simulink model "lcl_filter"  (R2022b)
settings: Solver=VariableStepAuto  StartTime=0.0  StopTime=10.0  RelTol=1e-3
libraries: spsSeriesRLCBranchLib x3, spsCurrentMeasurementLib x1, spsVoltageMeasurementLib x1
settings Model: Creator=nisha  LastModifiedBy=nisha

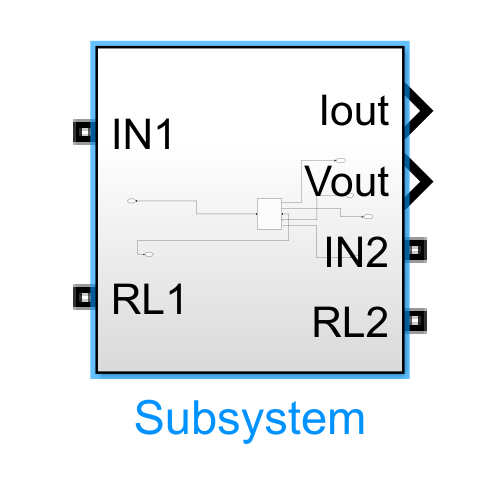
[thumbnail: Simulink's stored preview of the top-level diagram]
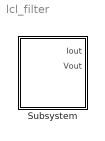
== system lcl_filter ==
  Subsystem : Subsystem

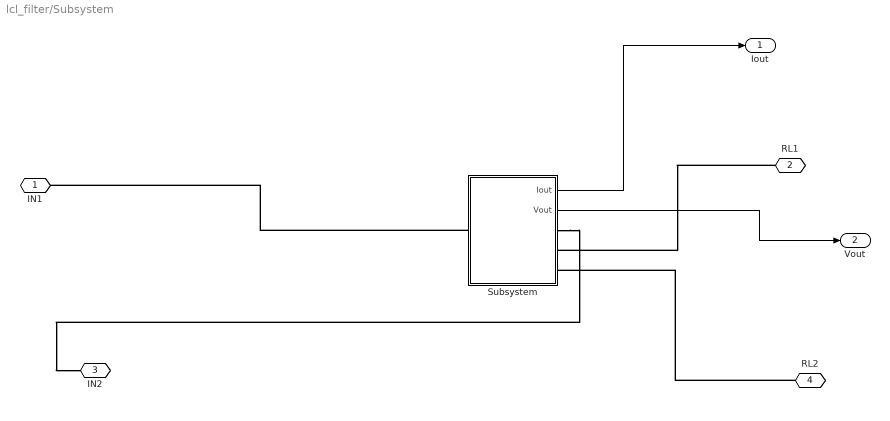
== system lcl_filter/Subsystem ==
  Subsystem : Subsystem
  "IN1 " : PMIOPort  Side=Left
  RL1 : PMIOPort  Port=2  Side=Left
  IN2 : PMIOPort  Port=3  Side=Right
  RL2 : PMIOPort  Port=4  Side=Right
  Iout : Outport
  Vout : Outport  Port=2
  wires:
  Subsystem/1(Iout) -> Iout/1
  Subsystem/2(Vout) -> Vout/1
  connections:
  Subsystem/LConn1 -- "IN1 "/RConn1
  Subsystem/RConn1 -- IN2/RConn1
  RL1/RConn1 -- Subsystem/RConn2
  RL2/RConn1 -- Subsystem/RConn3

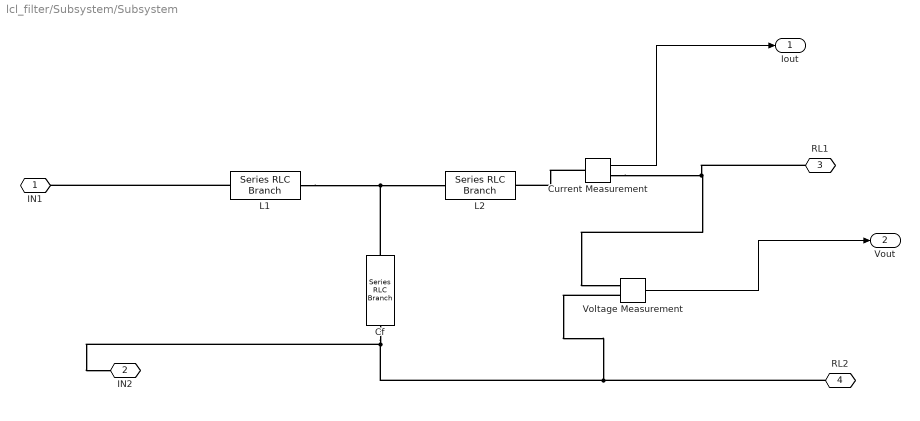
== system lcl_filter/Subsystem/Subsystem ==
  Cf : spsSeriesRLCBranchLib/Series RLC Branch  LConnTagsString=__new0  RConnTagsString=__new0  BranchType=C  Resistance=1e-3  Inductance=400e-3  SetiL0=off  InitialCurrent=0  Capacitance=680e-6  Setx0=off  InitialVoltage=0  Measurements=None
  Current Measurement : spsCurrentMeasurementLib/Current Measurement  PhasorSimulation=off  OutputType=Complex  PSBequivalent=0
  L1 : spsSeriesRLCBranchLib/Series RLC Branch  LConnTagsString=__new0  RConnTagsString=__new0  BranchType=L  Resistance=1e-3  Inductance=10e-3  SetiL0=off  InitialCurrent=0  Capacitance=1e-6  Setx0=off  InitialVoltage=0  Measurements=None
  L2 : spsSeriesRLCBranchLib/Series RLC Branch  LConnTagsString=__new0  RConnTagsString=__new0  BranchType=L  Resistance=1e-3  Inductance=10e-3  SetiL0=off  InitialCurrent=0  Capacitance=1e-6  Setx0=off  InitialVoltage=0  Measurements=None
  Voltage Measurement : spsVoltageMeasurementLib/Voltage Measurement  PhasorSimulation=off  OutputType=Complex  PSBequivalent=0
  IN1 : PMIOPort  Side=Left
  IN2 : PMIOPort  Port=2  Side=Right
  RL1 : PMIOPort  Port=3  Side=Right
  RL2 : PMIOPort  Port=4  Side=Right
  Iout : Outport
  Vout : Outport  Port=2
  wires:
  Voltage Measurement/1 -> Vout/1
  Current Measurement/1 -> Iout/1
  connections:
  Current Measurement/LConn1 -- L2/RConn1
  Current Measurement/RConn1 -- RL1/RConn1 -- Voltage Measurement/LConn1
  Cf/RConn1 -- IN2/RConn1 -- RL2/RConn1 -- Voltage Measurement/LConn2
  L1/RConn1 -- Cf/LConn1 -- L2/LConn1
  L1/LConn1 -- IN1/RConn1
